simulink library "outp"  (R2021b)
(part 3 of 10)

  bus_selector4/55 -> outpmodule/301(VDDM_ESC7NoComDTC_raw32)  "<VDDM_ESC7NoComDTC_raw32>"
  bus_selector2/24 -> outpmodule/39(VAPM_PASAFML_enum)  "<VAPM_PASAFML_enum>"
  outpmodule/569(VOUTP_V2BDCDCPosRlyFit_enum) -> bus_creator/569
  bus_selector2/23 -> outpmodule/38(VAPM_PASAFMR_enum)  "<VAPM_PASAFMR_enum>"
  bus_selector4/139 -> outpmodule/385(VDDM_LVSysErrPwrOutErr_flg)  "<VDDM_LVSysErrPwrOutErr_flg>"
  outpmodule/782(VOUTP_EMRC1ActMaxAvaEMRecpTrq_pct) -> bus_creator/782
  bus_selector6/16 -> outpmodule/417(VDID_HVESSCHARGELIM_kW)  "<VDID_HVESSCHARGELIM_kW>"
  outpmodule/179(VOUTP_DKCParkingModeCmd_enum) -> bus_creator/179
  outpmodule/454(VOUTP_AvgBattTempOFFR_C) -> bus_creator/454
  BACC_outputs/1 -> bus_selector1/1
  bus_selector2/93 -> outpmodule/108(VAPM_SASSpeedTimeOut_flg)  "<VAPM_SASSpeedTimeOut_flg>"
  outpmodule/487(VOUTP_AVGBATTEMPL_sec) -> bus_creator/487
  bus_selector2/99 -> outpmodule/114(VAPM_SASVTimeOut_flg)  "<VAPM_SASVTimeOut_flg>"
  bus_selector6/63 -> outpmodule/464(VDID_RESSTIMESOCPSARNGR_s)  "<VDID_RESSTIMESOCPSARNGR_s>"
  bus_selector2/95 -> outpmodule/110(VAPM_SASSpeedValidTimeOut_flg)  "<VAPM_SASSpeedValidTimeOut_flg>"
  bus_selector10/22 -> outpmodule/550(VPMM_LostHVComActivePwrDown_flg)  "<VPMM_LostHVComActivePwrDown_flg>"
  bus_selector2/91 -> outpmodule/106(VAPM_SASAngleTimeOut_flg)  "<VAPM_SASAngleTimeOut_flg>"
  bus_selector2/146 -> outpmodule/161(VAPM_IVIScreen_enum)  "<VAPM_IVIScreen_enum>"
  bus_selector2/14 -> outpmodule/29(VAPM_APSDRLR_cm)  "<VAPM_APSDRLR_cm>"
  outpmodule/466(VOUTP_RESSTIMESOCCHGRNGR_s) -> bus_creator/466
  bus_selector2/92 -> outpmodule/107(VAPM_SASSpeed_degps)  "<VAPM_SASSpeed_degps>"
  bus_selector4/19 -> outpmodule/265(VDDM_Lv4ErrDTC_raw32)  "<VDDM_Lv4ErrDTC_raw32>"
  bus_selector19/25 -> outpmodule/866(VVMC_FeatArbitrFinal_enum)  "<VVMC_FeatArbitrFinal_enum>"
  outpmodule/267(VOUTP_BrkSWNoBacDTC_raw32) -> bus_creator/267
  bus_selector2/90 -> outpmodule/105(VAPM_SASAngle_Deg)  "<VAPM_SASAngle_Deg>"
  bus_selector19/23 -> outpmodule/864(VVMC_ACCRequiredAccel_mps2)  "<VVMC_ACCRequiredAccel_mps2>"
  bus_selector6/22 -> outpmodule/423(VDID_PSAL_sec)  "<VDID_PSAL_sec>"
  bus_selector2/89 -> outpmodule/104(VAPM_EPSAOIControlTimeOut_flg)  "<VAPM_EPSAOIControlTimeOut_flg>"
  outpmodule/75(VOUTP_LFWhlRotDir_enum) -> bus_creator/75
  bus_selector3/45 -> outpmodule/235(VBCM_FDCBCMEmSVCmd_flg)  "<VBCM_FDCBCMEmSVCmd_flg>"
  bus_selector2/87 -> outpmodule/102(VAPM_DriIntendTimeOut_flg)  "<VAPM_DriIntendTimeOut_flg>"
  bus_selector16/83 -> outpmodule/828(VTQD_EMRC1DrvDemEMRtapTrq_pct)  "<VTQD_EMRC1DrvDemEMRtapTrq_pct>"
  outpmodule/295(VOUTP_APS1SigOoRDTC_raw32) -> bus_creator/295
  outpmodule/894(VOUTP_ADASLDWSta_enum) -> bus_creator/894
  bus_selector4/69 -> outpmodule/315(VDDM_RMLUSSDTC_raw32)  "<VDDM_RMLUSSDTC_raw32>"
  outpmodule/100(VOUTP_ShifterHandleCmdTimeOut_flg) -> bus_creator/100
  bus_selector2/88 -> outpmodule/103(VAPM_EPSAOIControl_enum)  "<VAPM_EPSAOIControl_enum>"
  bus_selector2/84 -> outpmodule/99(VAPM_ShifterHandleCmd_enum)  "<VAPM_ShifterHandleCmd_enum>"
  outpmodule/502(VOUTP_PCommandToBCM_enum) -> bus_creator/502
  bus_selector4/46 -> outpmodule/292(VDDM_TailgaSWDTC_raw32)  "<VDDM_TailgaSWDTC_raw32>"
  outpmodule/149(VOUTP_AVMparkingcancel_enum) -> bus_creator/149
  bus_selector2/86 -> outpmodule/101(VAPM_DriIntend_enum)  "<VAPM_DriIntend_enum>"
  bus_selector19/114 -> outpmodule/955(VVMC_FDCVMCMaxAngCtrlOutTqLim_Nm)  "<VVMC_FDCVMCMaxAngCtrlOutTqLim_Nm>"
  bus_selector2/82 -> outpmodule/97(VAPM_RRPulseCount_enum)  "<VAPM_RRPulseCount_enum>"
  outpmodule/815(VOUTP_RC1MaxRetSpdP2_rpm) -> bus_creator/815
  bus_selector2/81 -> outpmodule/96(VAPM_LRPulseCountTimeOut_flg)  "<VAPM_LRPulseCountTimeOut_flg>"
  bus_selector19/27 -> outpmodule/868(VVMC_LateralCtrl_flg)  "<VVMC_LateralCtrl_flg>"
  outpmodule/116(VOUTP_GRADETimeOut_flg) -> bus_creator/116
  bus_selector19/76 -> outpmodule/917(VVMC_LVDAACCStatusInformation_flg)  "<VVMC_LVDAACCStatusInformation_flg>"
  outpmodule/490(VOUTP_HEVMODE_enum) -> bus_creator/490
  outpmodule/725(VOUTP_WriteChkRRID_raw) -> bus_creator/725
  bus_selector2/80 -> outpmodule/95(VAPM_LRPulseCount_enum)  "<VAPM_LRPulseCount_enum>"
  bus_selector2/83 -> outpmodule/98(VAPM_RRPulseCountTimeOut_flg)  "<VAPM_RRPulseCountTimeOut_flg>"
  outpmodule/216(VOUTP_FDCBCMRDoorSta_flg) -> bus_creator/216
  outpmodule/809(VOUTP_EC1EMGainEndSpdGvn_gain) -> bus_creator/809
  bus_selector4/50 -> outpmodule/296(VDDM_APS2SigOoRDTC_raw32)  "<VDDM_APS2SigOoRDTC_raw32>"
  bus_selector2/79 -> outpmodule/94(VAPM_RFPulseCountTimeOut_flg)  "<VAPM_RFPulseCountTimeOut_flg>"
  bus_selector2/78 -> outpmodule/93(VAPM_RFPulseCount_enum)  "<VAPM_RFPulseCount_enum>"
  bus_selector19/40 -> outpmodule/881(VVMC_TimeGapLevel_enum)  "<VVMC_TimeGapLevel_enum>"
  bus_selector6/35 -> outpmodule/436(VDID_TEBPSAL_kWh)  "<VDID_TEBPSAL_kWh>"
  bus_selector15/80 -> outpmodule/728(VTPM_WriteChkfinLRID_raw)  "<VTPM_WriteChkfinLRID_raw>"
  bus_selector2/76 -> outpmodule/91(VAPM_LFPulseCount_enum)  "<VAPM_LFPulseCount_enum>"
  bus_selector13/17 -> outpmodule/621(VSYS_Variation_cnt)  "<VSYS_Variation_cnt>"
  bus_selector2/77 -> outpmodule/92(VAPM_LFPulseCountTimeOut_flg)  "<VAPM_LFPulseCountTimeOut_flg>"
  outpmodule/189(VOUTP_RAPSErrLv1_flg) -> bus_creator/189
  bus_selector3/18 -> outpmodule/208(VBCM_FDCBCMWasherCmd_flg)  "<VBCM_FDCBCMWasherCmd_flg>"
  bus_selector2/75 -> outpmodule/90(VAPM_RRPulseCountVTimeOut_flg)  "<VAPM_RRPulseCountVTimeOut_flg>"
  bus_selector2/140 -> outpmodule/155(VAPM_AVMErrSTA_flg)  "<VAPM_AVMErrSTA_flg>"
  outpmodule/187(VOUTP_APSPwrReq_enum) -> bus_creator/187
  bus_selector4/99 -> outpmodule/345(VDDM_MCUF1CSErrDTC_raw32)  "<VDDM_MCUF1CSErrDTC_raw32>"
  bus_selector6/52 -> outpmodule/453(VDID_AvgBattTempOVCL_C)  "<VDID_AvgBattTempOVCL_C>"
  bus_selector2/73 -> outpmodule/88(VAPM_LRPulseCountVTimeOut_flg)  "<VAPM_LRPulseCountVTimeOut_flg>"
  bus_selector2/70 -> outpmodule/85(VAPM_RFPulseCountV_flg)  "<VAPM_RFPulseCountV_flg>"
  outpmodule/864(VOUTP_ACCRequiredAccel_mps2) -> bus_creator/864
  outpmodule/106(VOUTP_SASAngleTimeOut_flg) -> bus_creator/106
  outpmodule/583(VOUTP_VSPTurnRight_enum) -> bus_creator/583
  bus_selector19/33 -> outpmodule/874(VVMC_ADASFaultSta_flg)  "<VVMC_ADASFaultSta_flg>"
  bus_selector2/71 -> outpmodule/86(VAPM_RFPulseCountVTimeOut_flg)  "<VAPM_RFPulseCountVTimeOut_flg>"
  outpmodule/609(VOUTP_CarModel2_cnt) -> bus_creator/609
  bus_selector4/123 -> outpmodule/369(VDDM_LFSensorFailDTC_raw32)  "<VDDM_LFSensorFailDTC_raw32>"
  outpmodule/137(VOUTP_ESCStandstill_flg) -> bus_creator/137
  bus_selector2/67 -> outpmodule/82(VAPM_RRWhlRotDirTimeOut_flg)  "<VAPM_RRWhlRotDirTimeOut_flg>"
  bus_selector9/1 -> outpmodule/517(VNMM_AllCANTxReq_flg)  "<VNMM_AllCANTxReq_flg>"
  bus_selector19/109 -> outpmodule/950(VVMC_FDCVMCAPSVRqEPSCtrl_flg)  "<VVMC_FDCVMCAPSVRqEPSCtrl_flg>"
  bus_selector4/105 -> outpmodule/351(VDDM_ESC1RCErrDTC_raw32)  "<VDDM_ESC1RCErrDTC_raw32>"
  bus_selector2/69 -> outpmodule/84(VAPM_LFPulseCountVTimeOut_flg)  "<VAPM_LFPulseCountVTimeOut_flg>"
  bus_selector2/68 -> outpmodule/83(VAPM_LFPulseCountV_flg)  "<VAPM_LFPulseCountV_flg>"
  bus_selector4/35 -> outpmodule/281(VDDM_MCUActDTC_raw32)  "<VDDM_MCUActDTC_raw32>"
  outpmodule/746(VOUTP_VCUMCUCtrlMdTQD_enum) -> bus_creator/746
  bus_selector19/59 -> outpmodule/900(VVMC_ADASCAMSpdLim_enum)  "<VVMC_ADASCAMSpdLim_enum>"
  bus_selector2/65 -> outpmodule/80(VAPM_LRWhlRotDirTimeOut_flg)  "<VAPM_LRWhlRotDirTimeOut_flg>"
  outpmodule/690(VOUTP_S1ID_raw32) -> bus_creator/690
  bus_selector10/24 -> outpmodule/552(VPMM_ChrgPowerUpFail_flg)  "<VPMM_ChrgPowerUpFail_flg>"
  bus_selector2/64 -> outpmodule/79(VAPM_LRWhlRotDir_enum)  "<VAPM_LRWhlRotDir_enum>"
  bus_selector19/57 -> outpmodule/898(VVMC_ACCTakeoverReq_flg)  "<VVMC_ACCTakeoverReq_flg>"
  bus_selector19/72 -> outpmodule/913(VVMC_LVDADisabled_flg)  "<VVMC_LVDADisabled_flg>"
  bus_selector2/66 -> outpmodule/81(VAPM_RRWhlRotDir_enum)  "<VAPM_RRWhlRotDir_enum>"
  bus_selector19/34 -> outpmodule/875(VVMC_AEBVehHoldReq_flg)  "<VVMC_AEBVehHoldReq_flg>"
  outpmodule/143(VOUTP_EPBExtApplyAvail_flg) -> bus_creator/143
  outpmodule/292(VOUTP_TailgaSWDTC_raw32) -> bus_creator/292
  outpmodule/481(VOUTP_BattTempPSAR_sec) -> bus_creator/481
  outpmodule/704(VOUTP_IDin_raw32) -> bus_creator/704
  bus_selector19/66 -> outpmodule/907(VVMC_ADASLaneModeR_enum)  "<VVMC_ADASLaneModeR_enum>"
  bus_selector2/62 -> outpmodule/77(VAPM_RFWhlRotDir_enum)  "<VAPM_RFWhlRotDir_enum>"
  bus_selector2/142 -> outpmodule/157(VAPM_IVIStatus_flg)  "<VAPM_IVIStatus_flg>"
  outpmodule/286(VOUTP_DrStSWDTC_raw32) -> bus_creator/286
  bus_selector4/73 -> outpmodule/319(VDDM_FLRUSSDTC_raw32)  "<VDDM_FLRUSSDTC_raw32>"
  outpmodule/211(VOUTP_FDCBCMRDRLCmd_flg) -> bus_creator/211
  bus_selector2/61 -> outpmodule/76(VAPM_LFWhlRotDirTimeOut_flg)  "<VAPM_LFWhlRotDirTimeOut_flg>"
  bus_selector2/57 -> outpmodule/72(VAPM_LRRawWhlSpeedVTimeOut_flg)  "<VAPM_LRRawWhlSpeedVTimeOut_flg>"
  bus_selector2/56 -> outpmodule/71(VAPM_LRRawWhlSpeedV_flg)  "<VAPM_LRRawWhlSpeedV_flg>"
  bus_selector6/18 -> outpmodule/419(VDID_HVESSENER_Whps)  "<VDID_HVESSENER_Whps>"
  bus_selector2/139 -> outpmodule/154(VAPM_AVMParkingmodeTimeOut_flg)  "<VAPM_AVMParkingmodeTimeOut_flg>"
  outpmodule/234(VOUTP_FDCBCMOSDrOpenSWSta_enum) -> bus_creator/234
  bus_selector16/73 -> outpmodule/818(VTQD_RC1PctTrqP3_pct)  "<VTQD_RC1PctTrqP3_pct>"
  bus_selector2/59 -> outpmodule/74(VAPM_RRRawWhlSpeedVTimeOut_flg)  "<VAPM_RRRawWhlSpeedVTimeOut_flg>"
  bus_selector2/60 -> outpmodule/75(VAPM_LFWhlRotDir_enum)  "<VAPM_LFWhlRotDir_enum>"
  outpmodule/166(VOUTP_TCSActiveTimeOut_flg) -> bus_creator/166
  outpmodule/532(VOUTP_ChrgState_enum) -> bus_creator/532
  BBCM_outputs/1 -> bus_selector3/1
  bus_selector10/27 -> outpmodule/555(VPMM_HVILDetectFail_flg)  "<VPMM_HVILDetectFail_flg>"
  bus_selector2/58 -> outpmodule/73(VAPM_RRRawWhlSpeedV_flg)  "<VAPM_RRRawWhlSpeedV_flg>"
  bus_selector2/166 -> outpmodule/181(VAPM_CAASVMCReqA_flg)  "<VAPM_CAASVMCReqA_flg>"
  bus_selector13/41 -> outpmodule/645(VSYS_ModelYear_cnt)  "<VSYS_ModelYear_cnt>"
  bus_selector4/108 -> outpmodule/354(VDDM_ESC5CSErrDTC_raw32)  "<VDDM_ESC5CSErrDTC_raw32>"
  bus_selector6/56 -> outpmodule/457(VDID_QTYPSATRIPSL_cnt)  "<VDID_QTYPSATRIPSL_cnt>"
  bus_selector2/72 -> outpmodule/87(VAPM_LRPulseCountV_flg)  "<VAPM_LRPulseCountV_flg>"
  outpmodule/227(VOUTP_FDCBCMFRoomLpSetSta_pct) -> bus_creator/227
  bus_selector12/6 -> outpmodule/595(VSCP_CFGEM1BAMPGN_raw)  "<VSCP_CFGEM1BAMPGN_raw>"
  bus_selector2/55 -> outpmodule/70(VAPM_RFRawWhlSpeedVTimeOut_flg)  "<VAPM_RFRawWhlSpeedVTimeOut_flg>"
  outpmodule/18(VOUTP_FSOffSw_enum) -> bus_creator/18
  outpmodule/611(VOUTP_ECU1_cnt) -> bus_creator/611
  bus_selector4/148 -> outpmodule/394(VDDM_VCUHoodSWSta_flg)  "<VDDM_VCUHoodSWSta_flg>"
  bus_selector2/51 -> outpmodule/66(VAPM_RRRawWhlSpeedTimeOut_flg)  "<VAPM_RRRawWhlSpeedTimeOut_flg>"
  bus_selector6/33 -> outpmodule/434(VDID_TNECPSAL_kWh)  "<VDID_TNECPSAL_kWh>"
  bus_selector3/13 -> outpmodule/203(VBCM_FDCBCMStopINDCmd_flg)  "<VBCM_FDCBCMStopINDCmd_flg>"
  outpmodule/784(VOUTP_EC1PercTorqIdleP1_pct) -> bus_creator/784
  bus_selector2/50 -> outpmodule/65(VAPM_RRRawWhlSpeed_kph)  "<VAPM_RRRawWhlSpeed_kph>"
  bus_selector2/31 -> outpmodule/46(VAPM_USSStaRCL_flg)  "<VAPM_USSStaRCL_flg>"
  bus_selector2/22 -> outpmodule/37(VAPM_PASARCL_enum)  "<VAPM_PASARCL_enum>"
  bus_selector16/53 -> outpmodule/798(VTQD_EC1EMReqSpdCtrlUpLmt_rpm)  "<VTQD_EC1EMReqSpdCtrlUpLmt_rpm>"
  bus_selector3/16 -> outpmodule/206(VBCM_FDCBCMCallBellCmd_flg)  "<VBCM_FDCBCMCallBellCmd_flg>"
  bus_selector2/20 -> outpmodule/35(VAPM_PASARML_enum)  "<VAPM_PASARML_enum>"
  bus_selector19/101 -> outpmodule/942(VVMC_CAASActive_flg)  "<VVMC_CAASActive_flg>"
  outpmodule/850(VOUTP_FeatArbitrSta_enum) -> bus_creator/850
  bus_selector6/30 -> outpmodule/431(VDID_TNBCPSAR_Ahr)  "<VDID_TNBCPSAR_Ahr>"
  bus_selector16/81 -> outpmodule/826(VTQD_ETC1ShiftrPgs_enum)  "<VTQD_ETC1ShiftrPgs_enum>"
  bus_selector2/46 -> outpmodule/61(VAPM_RFRawWhlSpeed_kph)  "<VAPM_RFRawWhlSpeed_kph>"
  outpmodule/773(VOUTP_EEC3NFricPercTorq_pct) -> bus_creator/773
  bus_selector2/36 -> outpmodule/51(VAPM_USSStaFCR_flg)  "<VAPM_USSStaFCR_flg>"
  bus_selector2/103 -> outpmodule/118(VAPM_YawRateTimeOut_flg)  "<VAPM_YawRateTimeOut_flg>"
  bus_selector2/28 -> outpmodule/43(VAPM_USSStaRLR_flg)  "<VAPM_USSStaRLR_flg>"
  bus_selector4/63 -> outpmodule/309(VDDM_DiagRRTSDTC_raw32)  "<VDDM_DiagRRTSDTC_raw32>"
  bus_selector3/49 -> outpmodule/239(VBCM_FDCBCMMDCloseSVCmd_flg)  "<VBCM_FDCBCMMDCloseSVCmd_flg>"
  outpmodule/241(VOUTP_FDCBCMRTurnSWSta_flg) -> bus_creator/241
  bus_selector2/101 -> outpmodule/116(VAPM_GRADETimeOut_flg)  "<VAPM_GRADETimeOut_flg>"
  bus_selector16/64 -> outpmodule/809(VTQD_EC1EMGainEndSpdGvn_gain)  "<VTQD_EC1EMGainEndSpdGvn_gain>"
  bus_selector2/49 -> outpmodule/64(VAPM_LRRawWhlSpeedTimeOut_flg)  "<VAPM_LRRawWhlSpeedTimeOut_flg>"
  bus_selector2/159 -> outpmodule/174(VAPM_APSAngleTarget_Deg)  "<VAPM_APSAngleTarget_Deg>"
  bus_selector2/53 -> outpmodule/68(VAPM_LFRawWhlSpeedVTimeOut_flg)  "<VAPM_LFRawWhlSpeedVTimeOut_flg>"
  outpmodule/432(VOUTP_TNBCPSAL_Ahr) -> bus_creator/432
  bus_selector4/20 -> outpmodule/266(VDDM_BrkSWErrDTC_raw32)  "<VDDM_BrkSWErrDTC_raw32>"
  bus_selector3/56 -> outpmodule/246(VBCM_KeepWakeUp_flg)  "<VBCM_KeepWakeUp_flg>"
  outpmodule/906(VOUTP_ADASLaneModeL_enum) -> bus_creator/906
  outpmodule/20(VOUTP_ChrgPlugSta_enum) -> bus_creator/20
  bus_selector2/54 -> outpmodule/69(VAPM_RFRawWhlSpeedV_flg)  "<VAPM_RFRawWhlSpeedV_flg>"
  bus_selector10/20 -> outpmodule/548(VPMM_VCUMCUFailRst_flg)  "<VPMM_VCUMCUFailRst_flg>"
  bus_selector2/112 -> outpmodule/127(VAPM_LatAccelV_flg)  "<VAPM_LatAccelV_flg>"
  bus_selector1/8 -> outpmodule/8(VACC_EHPSMotorDemSpd_rpm)  "<VACC_EHPSMotorDemSpd_rpm>"
  outpmodule/359(VOUTP_LRBatwarnDTC_raw32) -> bus_creator/359
  outpmodule/61(VOUTP_RFRawWhlSpeed_kph) -> bus_creator/61
  bus_selector2/113 -> outpmodule/128(VAPM_LatAccelVTimeOut_flg)  "<VAPM_LatAccelVTimeOut_flg>"
  bus_selector10/44 -> outpmodule/572(VPMM_V2BAux2RlySta_enum)  "<VPMM_V2BAux2RlySta_enum>"
  BAPM_outputs/1 -> bus_selector2/1
  outpmodule/228(VOUTP_FDCBCMFRoomLpCmd_pct) -> bus_creator/228
  outpmodule/249(VOUTP_C3BMS6LCDTC_raw32) -> bus_creator/249
  bus_selector6/72 -> outpmodule/473(VDID_PROTOCOLID_enum)  "<VDID_PROTOCOLID_enum>"
  bus_selector2/6 -> outpmodule/21(VAPM_PASDRMR_cm)  "<VAPM_PASDRMR_cm>"
  outpmodule/865(VOUTP_DISCReqAcc_mps2) -> bus_creator/865
  bus_selector2/121 -> outpmodule/136(VAPM_BrkSwVTimeOut_flg)  "<VAPM_BrkSwVTimeOut_flg>"
  outpmodule/349(VOUTP_ESC7RCErrDTC_raw32) -> bus_creator/349
  outpmodule/60(VOUTP_LFRawWhlSpeedTimeOut_flg) -> bus_creator/60
  bus_selector4/65 -> outpmodule/311(VDDM_FMLUSSDTC_raw32)  "<VDDM_FMLUSSDTC_raw32>"
  bus_selector2/4 -> outpmodule/19(VAPM_FSOffSwTimeOut_flg)  "<VAPM_FSOffSwTimeOut_flg>"
  outpmodule/277(VOUTP_MidLvSaChkDTC_raw32) -> bus_creator/277
  outpmodule/464(VOUTP_RESSTIMESOCPSARNGR_s) -> bus_creator/464
  bus_selector3/40 -> outpmodule/230(VBCM_FDCBCMMRoomLpCmd_pct)  "<VBCM_FDCBCMMRoomLpCmd_pct>"
  bus_selector2/39 -> outpmodule/54(VAPM_SNSRLayout_enum)  "<VAPM_SNSRLayout_enum>"
  outpmodule/59(VOUTP_LFRawWhlSpeed_kph) -> bus_creator/59
  bus_selector10/43 -> outpmodule/571(VPMM_V2BAux1RlyFit_enum)  "<VPMM_V2BAux1RlyFit_enum>"
  outpmodule/385(VOUTP_LVSysErrPwrOutErr_flg) -> bus_creator/385
  bus_selector6/27 -> outpmodule/428(VDID_HVBNAH_Ahr)  "<VDID_HVBNAH_Ahr>"
  bus_selector2/74 -> outpmodule/89(VAPM_RRPulseCountV_flg)  "<VAPM_RRPulseCountV_flg>"
  bus_selector6/29 -> outpmodule/430(VDID_IGNCNTR_cnt)  "<VDID_IGNCNTR_cnt>"
  bus_selector2/160 -> outpmodule/175(VAPM_APSVRqEPASCtrl_flg)  "<VAPM_APSVRqEPASCtrl_flg>"
  outpmodule/84(VOUTP_LFPulseCountVTimeOut_flg) -> bus_creator/84
  outpmodule/651(VOUTP_LRBatWarn_flg) -> bus_creator/651
  bus_selector3/34 -> outpmodule/224(VBCM_FDCBCMInnerBuzzerCmd_flg)  "<VBCM_FDCBCMInnerBuzzerCmd_flg>"
  bus_selector10/55 -> outpmodule/583(VPMM_VSPTurnRight_enum)  "<VPMM_VSPTurnRight_enum>"
  outpmodule/897(VOUTP_ForceLowBeam_enum) -> bus_creator/897
  bus_selector4/104 -> outpmodule/350(VDDM_ESC7CSErrDTC_raw32)  "<VDDM_ESC7CSErrDTC_raw32>"
  bus_selector19/85 -> outpmodule/926(VVMC_FCMLDWFault_flg)  "<VVMC_FCMLDWFault_flg>"
  outpmodule/534(VOUTP_PowerDownFault_enum) -> bus_creator/534
  bus_selector2/94 -> outpmodule/109(VAPM_SASSpeedValid_flg)  "<VAPM_SASSpeedValid_flg>"
  outpmodule/391(VOUTP_VCURLDoorSta_flg) -> bus_creator/391
  bus_selector19/17 -> outpmodule/858(VVMC_SafetyCtrl_flg)  "<VVMC_SafetyCtrl_flg>"
  bus_selector4/17 -> outpmodule/263(VDDM_Lv2ErrDTC_raw32)  "<VDDM_Lv2ErrDTC_raw32>"
  outpmodule/786(VOUTP_EC1PercTorqIdleP2_pct) -> bus_creator/786
  BTHC_outputs/1 -> bus_selector14/1
  bus_selector1/4 -> outpmodule/4(VACC_CACPresReady_flg)  "<VACC_CACPresReady_flg>"
  bus_selector2/37 -> outpmodule/52(VAPM_USSStaFCL_flg)  "<VAPM_USSStaFCL_flg>"
  bus_selector6/11 -> outpmodule/412(VDID_HEVBATT_V)  "<VDID_HEVBATT_V>"
  bus_selector2/174 -> outpmodule/189(VAPM_RAPSErrLv1_flg)  "<VAPM_RAPSErrLv1_flg>"
  outpmodule/210(VOUTP_FDCBCMLDRLCmd_flg) -> bus_creator/210
  bus_selector6/12 -> outpmodule/413(VDID_ODOMETER_km)  "<VDID_ODOMETER_km>"
  bus_selector2/115 -> outpmodule/130(VAPM_LongAccelVTimeOut_flg)  "<VAPM_LongAccelVTimeOut_flg>"
  bus_selector6/25 -> outpmodule/426(VDID_CPSAR_sec)  "<VDID_CPSAR_sec>"
  bus_selector3/20 -> outpmodule/210(VBCM_FDCBCMLDRLCmd_flg)  "<VBCM_FDCBCMLDRLCmd_flg>"
  bus_selector2/85 -> outpmodule/100(VAPM_ShifterHandleCmdTimeOut_flg)  "<VAPM_ShifterHandleCmdTimeOut_flg>"
  bus_selector4/79 -> outpmodule/325(VDDM_FCM3NoComDTC_raw32)  "<VDDM_FCM3NoComDTC_raw32>"
  bus_selector13/21 -> outpmodule/625(VSYS_Dash2_cnt)  "<VSYS_Dash2_cnt>"
  bus_selector4/121 -> outpmodule/367(VDDM_LRWheelTmpHighDTC_raw32)  "<VDDM_LRWheelTmpHighDTC_raw32>"
  bus_selector6/6 -> outpmodule/407(VDID_APPD_pct)  "<VDID_APPD_pct>"
  outpmodule/517(VOUTP_AllCANTxReq_flg) -> bus_creator/517
  bus_selector2/44 -> outpmodule/59(VAPM_LFRawWhlSpeed_kph)  "<VAPM_LFRawWhlSpeed_kph>"
  bus_selector19/68 -> outpmodule/909(VVMC_ADASISASta_enum)  "<VVMC_ADASISASta_enum>"
  bus_selector6/7 -> outpmodule/408(VDID_APPE_pct)  "<VDID_APPE_pct>"
  outpmodule/338(VOUTP_ACCAccelCmdErrDetDTC_raw32) -> bus_creator/338
  bus_selector2/96 -> outpmodule/111(VAPM_SASCAL_flg)  "<VAPM_SASCAL_flg>"
  bus_selector2/150 -> outpmodule/165(VAPM_TCSActive_flg)  "<VAPM_TCSActive_flg>"
  outpmodule/82(VOUTP_RRWhlRotDirTimeOut_flg) -> bus_creator/82
  bus_selector6/4 -> outpmodule/405(VDID_WARMUPS_cnt)  "<VDID_WARMUPS_cnt>"
  bus_selector3/53 -> outpmodule/243(VBCM_FDCBCMBrakeCmd_flg)  "<VBCM_FDCBCMBrakeCmd_flg>"
  outpmodule/118(VOUTP_YawRateTimeOut_flg) -> bus_creator/118
  bus_selector6/9 -> outpmodule/410(VDID_CLRTIME_min)  "<VDID_CLRTIME_min>"
  outpmodule/668(VOUTP_RRWheelDebug_flg) -> bus_creator/668
  bus_selector6/80 -> outpmodule/481(VDID_BattTempPSAR_sec)  "<VDID_BattTempPSAR_sec>"
  bus_selector4/9 -> outpmodule/255(VDDM_C3CCU1LCDTC_raw32)  "<VDDM_C3CCU1LCDTC_raw32>"
  bus_selector15/89 -> outpmodule/737(VTPM_FlashS3ID_raw)  "<VTPM_FlashS3ID_raw>"
  bus_selector6/1 -> outpmodule/402(VDID_VSS_kph)  "<VDID_VSS_kph>"
  outpmodule/825(VOUTP_TUpAIND_enum) -> bus_creator/825
  bus_selector8/4 -> outpmodule/516(VDSC_DISCButtSta_flg)  "<VDSC_DISCButtSta_flg>"
  outpmodule/492(VOUTP_DIDModelVersion_raw) -> bus_creator/492
  outpmodule/65(VOUTP_RRRawWhlSpeed_kph) -> bus_creator/65
  bus_selector4/91 -> outpmodule/337(VDDM_CCUSigErrDetDTC_raw32)  "<VDDM_CCUSigErrDetDTC_raw32>"
  bus_selector4/34 -> outpmodule/280(VDDM_HVRlyOpDTC_raw32)  "<VDDM_HVRlyOpDTC_raw32>"
  bus_selector19/56 -> outpmodule/897(VVMC_ForceLowBeam_enum)  "<VVMC_ForceLowBeam_enum>"
  bus_selector10/57 -> outpmodule/585(VPMM_FogTMSRlyCMD_enum)  "<VPMM_FogTMSRlyCMD_enum>"
  bus_selector6/5 -> outpmodule/406(VDID_CLRDIST_km)  "<VDID_CLRDIST_km>"
  outpmodule/919(VOUTP_FCMACCmode_enum) -> bus_creator/919
  bus_selector2/129 -> outpmodule/144(VAPM_EPBExtApplyAvailTimeOut_flg)  "<VAPM_EPBExtApplyAvailTimeOut_flg>"
  bus_selector3/5 -> outpmodule/195(VBCM_FDCBCMSMKRCmd_flg)  "<VBCM_FDCBCMSMKRCmd_flg>"
  bus_selector2/100 -> outpmodule/115(VAPM_GRADE_Deg)  "<VAPM_GRADE_Deg>"
  bus_selector4/28 -> outpmodule/274(VDDM_BMSRdyDTC_raw32)  "<VDDM_BMSRdyDTC_raw32>"
  bus_selector13/2 -> outpmodule/606(VSYS_HWVer2_cnt)  "<VSYS_HWVer2_cnt>"
  bus_selector2/133 -> outpmodule/148(VAPM_EPBStaTimeOut_flg)  "<VAPM_EPBStaTimeOut_flg>"
  bus_selector2/52 -> outpmodule/67(VAPM_LFRawWhlSpeedV_flg)  "<VAPM_LFRawWhlSpeedV_flg>"
  bus_selector6/28 -> outpmodule/429(VDID_HVBNE_kWh)  "<VDID_HVBNE_kWh>"
  bus_selector2/172 -> outpmodule/187(VAPM_APSPwrReq_enum)  "<VAPM_APSPwrReq_enum>"
  outpmodule/206(VOUTP_FDCBCMCallBellCmd_flg) -> bus_creator/206
  bus_selector4/30 -> outpmodule/276(VDDM_HiLvSaChkDTC_raw32)  "<VDDM_HiLvSaChkDTC_raw32>"
  bus_selector15/96 -> outpmodule/744(VTPM_ModelVersion_raw)  "<VTPM_ModelVersion_raw>"
  bus_selector16/30 -> outpmodule/775(VTQD_ETC2ActDriveDirect_enum)  "<VTQD_ETC2ActDriveDirect_enum>"
  bus_selector7/18 -> outpmodule/511(VDKC_FDCDKCAllowSleep_flg)  "<VDKC_FDCDKCAllowSleep_flg>"
  bus_selector4/6 -> outpmodule/252(VDDM_C3BMS1LCDTC_raw32)  "<VDDM_C3BMS1LCDTC_raw32>"
  outpmodule/85(VOUTP_RFPulseCountV_flg) -> bus_creator/85
  outpmodule/684(VOUTP_CWheelTips_enum) -> bus_creator/684
  bus_selector15/81 -> outpmodule/729(VTPM_WriteChkfinRRID_raw)  "<VTPM_WriteChkfinRRID_raw>"
  BDKC_outputs/1 -> bus_selector7/1
  bus_selector4/27 -> outpmodule/273(VDDM_HVRlyCloDTC_raw32)  "<VDDM_HVRlyCloDTC_raw32>"
  bus_selector1/6 -> outpmodule/6(VACC_CACOverrun_flg)  "<VACC_CACOverrun_flg>"
  bus_selector15/20 -> outpmodule/668(VTPM_RRWheelDebug_flg)  "<VTPM_RRWheelDebug_flg>"
  outpmodule/69(VOUTP_RFRawWhlSpeedV_flg) -> bus_creator/69
  bus_selector2/105 -> outpmodule/120(VAPM_LatAccelTimeOut_flg)  "<VAPM_LatAccelTimeOut_flg>"
  bus_selector19/10 -> outpmodule/851(VVMC_FeatReqSpd_kph)  "<VVMC_FeatReqSpd_kph>"
  bus_selector4/26 -> outpmodule/272(VDDM_DCDC4PreDTC_raw32)  "<VDDM_DCDC4PreDTC_raw32>"
  outpmodule/953(VOUTP_FDCVMCAngCtrlTqWtGn_pct) -> bus_creator/953
  outpmodule/68(VOUTP_LFRawWhlSpeedVTimeOut_flg) -> bus_creator/68
  bus_selector6/8 -> outpmodule/409(VDID_MILTIME_min)  "<VDID_MILTIME_min>"
  bus_selector2/155 -> outpmodule/170(VAPM_APSRQDisplay_enum)  "<VAPM_APSRQDisplay_enum>"
  bus_selector4/38 -> outpmodule/284(VDDM_LVSupLoDTC_raw32)  "<VDDM_LVSupLoDTC_raw32>"
  bus_selector2/47 -> outpmodule/62(VAPM_RFRawWhlSpeedTimeOut_flg)  "<VAPM_RFRawWhlSpeedTimeOut_flg>"
  outpmodule/163(VOUTP_ABSActive_flg) -> bus_creator/163
  outpmodule/513(VOUTP_DISCTurn_flg) -> bus_creator/513
  bus_selector2/40 -> outpmodule/55(VAPM_StaFSya_flg)  "<VAPM_StaFSya_flg>"
  bus_selector19/98 -> outpmodule/939(VVMC_CCMSASpdWar_flg)  "<VVMC_CCMSASpdWar_flg>"
  bus_selector12/10 -> outpmodule/599(VSCP_DTbyte2_raw)  "<VSCP_DTbyte2_raw>"
  bus_selector4/114 -> outpmodule/360(VDDM_RRBatwarnDTC_raw32)  "<VDDM_RRBatwarnDTC_raw32>"
  bus_selector8/2 -> outpmodule/514(VDSC_DISCTargetSpd_kph)  "<VDSC_DISCTargetSpd_kph>"
  bus_selector19/35 -> outpmodule/876(VVMC_ACCVehHoldReq_flg)  "<VVMC_ACCVehHoldReq_flg>"
  outpmodule/944(VOUTP_CalibratedAccX_G) -> bus_creator/944
  bus_selector2/41 -> outpmodule/56(VAPM_ModOperation_enum)  "<VAPM_ModOperation_enum>"
  bus_selector9/11 -> outpmodule/527(VNMM_SysNMmSta_enum)  "<VNMM_SysNMmSta_enum>"
  bus_selector2/167 -> outpmodule/182(VAPM_APSShiftPosnReq_enum)  "<VAPM_APSShiftPosnReq_enum>"
  outpmodule/177(VOUTP_CAASSta_enum) -> bus_creator/177
  outpmodule/73(VOUTP_RRRawWhlSpeedV_flg) -> bus_creator/73
  outpmodule/493(VOUTP_DIDModelVersionChksum_raw) -> bus_creator/493
  bus_selector6/2 -> outpmodule/403(VDID_RUNTM_s)  "<VDID_RUNTM_s>"
  bus_selector4/54 -> outpmodule/300(VDDM_Shifter1NoComDTC_raw32)  "<VDDM_Shifter1NoComDTC_raw32>"
  outpmodule/742(VOUTP_LProgress_enum) -> bus_creator/742
  bus_selector6/3 -> outpmodule/404(VDID_MILDIST_km)  "<VDID_MILDIST_km>"
  bus_selector12/3 -> outpmodule/592(VSCP_CFGEM1BAMTSize_raw)  "<VSCP_CFGEM1BAMTSize_raw>"
  bus_selector16/61 -> outpmodule/806(VTQD_EC1EMSupTSC1CtrlPG2_cnt)  "<VTQD_EC1EMSupTSC1CtrlPG2_cnt>"
  bus_selector3/19 -> outpmodule/209(VBCM_FDCBCMWiperLCmd_flg)  "<VBCM_FDCBCMWiperLCmd_flg>"
  bus_selector19/81 -> outpmodule/922(VVMC_ADASLanecurveL_raw32)  "<VVMC_ADASLanecurveL_raw32>"
  bus_selector4/76 -> outpmodule/322(VDDM_FCM2NoComDTC_raw32)  "<VDDM_FCM2NoComDTC_raw32>"
  bus_selector2/45 -> outpmodule/60(VAPM_LFRawWhlSpeedTimeOut_flg)  "<VAPM_LFRawWhlSpeedTimeOut_flg>"
  outpmodule/565(VOUTP_V2BAirPosRlyFit_enum) -> bus_creator/565
  outpmodule/921(VOUTP_ADASLanetypeL_enum) -> bus_creator/921
  bus_selector2/98 -> outpmodule/113(VAPM_SASV_flg)  "<VAPM_SASV_flg>"
  outpmodule/305(VOUTP_DiagHCrashDTC_raw32) -> bus_creator/305
  bus_selector9/5 -> outpmodule/521(VNMM_ErrorState_enum)  "<VNMM_ErrorState_enum>"
  bus_selector2/63 -> outpmodule/78(VAPM_RFWhlRotDirTimeOut_flg)  "<VAPM_RFWhlRotDirTimeOut_flg>"
  bus_selector16/85 -> outpmodule/830(VTQD_EMRC1SACtrlDev_cnt)  "<VTQD_EMRC1SACtrlDev_cnt>"
  bus_selector2/26 -> outpmodule/41(VAPM_USSStaRMR_flg)  "<VAPM_USSStaRMR_flg>"
  bus_selector3/28 -> outpmodule/218(VBCM_FDCBCMLBSDRCmd_flg)  "<VBCM_FDCBCMLBSDRCmd_flg>"
  outpmodule/62(VOUTP_RFRawWhlSpeedTimeOut_flg) -> bus_creator/62
  bus_selector4/25 -> outpmodule/271(VDDM_MCU4PreDTC_raw32)  "<VDDM_MCU4PreDTC_raw32>"
  outpmodule/254(VOUTP_C3CCU1CSDTC_raw32) -> bus_creator/254
  bus_selector15/64 -> outpmodule/712(VTPM_ID4messageALTU_raw8)  "<VTPM_ID4messageALTU_raw8>"
  bus_selector16/54 -> outpmodule/799(VTQD_EC1EMReqTrqCtrlUpLmt_pct)  "<VTQD_EC1EMReqTrqCtrlUpLmt_pct>"
  outpmodule/64(VOUTP_LRRawWhlSpeedTimeOut_flg) -> bus_creator/64
  bus_selector2/21 -> outpmodule/36(VAPM_PASARCR_enum)  "<VAPM_PASARCR_enum>"
  bus_selector6/78 -> outpmodule/479(VDID_PKERNumerator_kphsqr)  "<VDID_PKERNumerator_kphsqr>"
  bus_selector19/1 -> outpmodule/842(VVMC_FeatSetSpdFinal_raw32)  "<VVMC_FeatSetSpdFinal_raw32>"
  bus_selector3/30 -> outpmodule/220(VBCM_FDCBCMRBSDRCmd_flg)  "<VBCM_FDCBCMRBSDRCmd_flg>"
  outpmodule/66(VOUTP_RRRawWhlSpeedTimeOut_flg) -> bus_creator/66
  bus_selector13/39 -> outpmodule/643(VSYS_PmicBootPath_raw32)  "<VSYS_PmicBootPath_raw32>"
  bus_selector4/47 -> outpmodule/293(VDDM_EDriveSysErrVCUErr_flg)  "<VDDM_EDriveSysErrVCUErr_flg>"
  bus_selector2/102 -> outpmodule/117(VAPM_YawRate_degps)  "<VAPM_YawRate_degps>"
  bus_selector2/34 -> outpmodule/49(VAPM_USSStaFLR_flg)  "<VAPM_USSStaFLR_flg>"
  bus_selector19/41 -> outpmodule/882(VVMC_ACCJerkUpperLimit_mps3)  "<VVMC_ACCJerkUpperLimit_mps3>"
  outpmodule/529(VOUTP_SysPowerMode_enum) -> bus_creator/529
  bus_selector13/30 -> outpmodule/634(VSYS_NvWriteReqRisingEdge_flg)  "<VSYS_NvWriteReqRisingEdge_flg>"
  outpmodule/67(VOUTP_LFRawWhlSpeedV_flg) -> bus_creator/67
  bus_selector6/92 -> outpmodule/493(VDID_DIDModelVersionChksum_raw)  "<VDID_DIDModelVersionChksum_raw>"
  outpmodule/159(VOUTP_CAASSw_enum) -> bus_creator/159
  outpmodule/71(VOUTP_LRRawWhlSpeedV_flg) -> bus_creator/71
  bus_selector15/47 -> outpmodule/695(VTPM_S2L_enum)  "<VTPM_S2L_enum>"
  outpmodule/698(VOUTP_ALFin_flg) -> bus_creator/698
  outpmodule/156(VOUTP_AVMErrSTATimeOut_flg) -> bus_creator/156
  bus_selector4/61 -> outpmodule/307(VDDM_DiagFRTSDTC_raw32)  "<VDDM_DiagFRTSDTC_raw32>"
  outpmodule/58(VOUTP_BrkPedalPosTimeOut_flg) -> bus_creator/58
  bus_selector13/26 -> outpmodule/630(VSYS_SHA5_cnt)  "<VSYS_SHA5_cnt>"
  outpmodule/711(VOUTP_ID3messageALTU_raw8) -> bus_creator/711
  outpmodule/63(VOUTP_LRRawWhlSpeed_kph) -> bus_creator/63
  bus_selector9/10 -> outpmodule/526(VNMM_ActiveWU_flg)  "<VNMM_ActiveWU_flg>"
  bus_selector2/97 -> outpmodule/112(VAPM_SASCALTimeOut_flg)  "<VAPM_SASCALTimeOut_flg>"
  outpmodule/460(VOUTP_ETMATOER_kWh) -> bus_creator/460
  bus_selector6/10 -> outpmodule/411(VDID_BATSOC_pct)  "<VDID_BATSOC_pct>"
  bus_selector19/70 -> outpmodule/911(VVMC_ADASFCWMute_flg)  "<VVMC_ADASFCWMute_flg>"
  outpmodule/463(VOUTP_ETMBTOEL_kWh) -> bus_creator/463
  outpmodule/945(VOUTP_CalibratedAccY_G) -> bus_creator/945
  Constant/1 -> outpmodule/15(VACC_CACFanReq_flg)
